simulink model "qbot_platform_obstacle_detection"  (R2023a)
settings: Solver=ode1  StartTime=0.0  StopTime=inf  FixedStep=1/30  RelTol=1e-3  EnableMultiTasking=on
InitFcn:
  | theta = linspace(pi/2, pi/4, 52);
  | theta_p = pi/2 - theta;
  | first = 1./cos(theta_p);
  | middle = first(end).*ones(1, 106);
  | last = flip(first);
  | 
  | zone = [first, middle, last]';
model workspace (MAT data in the model file):
  downCamStepSize = Simulink.Parameter
  downCamStepSize.Value = Simulink.data.Expression
  downCamStepSize.Value.ExpressionString = "qc_get_step_size*ceil(1/30/qc_get_step_size)"
  downCamStepSize.DataType = 'auto'
  downCamStepSize.Complexity = 'real'
  downCamStepSize.Dimensions = -1
  lidarStepSize = Simulink.Parameter
  lidarStepSize.Value = Simulink.data.Expression
  lidarStepSize.Value.ExpressionString = "qc_get_step_size*ceil(1/5/qc_get_step_size)"
  lidarStepSize.DataType = 'auto'
  lidarStepSize.Complexity = 'real'
  lidarStepSize.Dimensions = -1
  mainStepSize = Simulink.Parameter
  mainStepSize.Value = Simulink.data.Expression
  mainStepSize.Value.ExpressionString = "qc_get_step_size"
  mainStepSize.DataType = 'auto'
  mainStepSize.Complexity = 'real'
  mainStepSize.Dimensions = -1
  realSenseStepSize = Simulink.Parameter
  realSenseStepSize.Value = Simulink.data.Expression
  realSenseStepSize.Value.ExpressionString = "qc_get_step_size*ceil(1/30/qc_get_step_size)"
  realSenseStepSize.DataType = 'auto'
  realSenseStepSize.Complexity = 'real'
  realSenseStepSize.Dimensions = -1
undefined symbols (not defined in the file): Point, qc_get_step_size
libraries: quarc_library x12, simulink x2
settings Model: SimulationMode=external  ExtModeTrigDuration=10000  Creator=mbohra  LastModifiedBy=mbohra
settings SolverCC: AlgebraicLoopSolver=TrustRegion  PositivePriorityOrder=on
settings DataIOCC: ReturnWorkspaceOutputs=off
settings DebuggingCC: UnconnectedInputMsg=warning  UnconnectedOutputMsg=warning  UnconnectedLineMsg=warning  ArithmeticOperatorsInVariantConditions=warning
settings HardwareCC: ProdBitPerLong=64  ProdLargestAtomicInteger=LongLong  ProdLargestAtomicFloat=Double  ProdLongLongMode=on  ProdHWDeviceType=ARM Compatible->ARM 64-bit (LP64)
settings ModelReferenceCC: EnableRefExpFcnMdlSchedulingChecks=on
settings SFSimCC: SimUseLocalCustomCode=off  CustomCodeUndefinedFunction=UseInterfaceOnly
settings RTWCC: Description=QUARC Linux Raspberry Pi Arm64 Target (QBot Platform Alpha) Using Toolchain  SystemTargetFile=quarc_linux_pi_arm64.tlc  TemplateMakefile=quarc_default_tmf  RTWUseLocalCustomCode=off  Toolchain=QUARC linux_pi_arm64 | gmake (64-bit Windows)  BuildConfiguration=Faster Runs
settings CodeAppCC: StateflowObjectComments=on
settings STFCustomTargetCC: SystemTargetFile=quarc_linux_pi_arm64.tlc
settings GRTTargetCC: ParMdlRefBuildCompliant=off  CompOptLevelCompliant=off  CombineOutputUpdateFcns=off  MatFileLogging=off  CPPClassGenCompliant=off  GRTInterface=on  ExtMode=on  ExtModeMexFile=quarc_comm  ExtModeMexArgs='-w -d /tmp -uri %u','tcpip://192.168.2.80:17001'
settings ConfigComp: CovMetricSettings=dswe

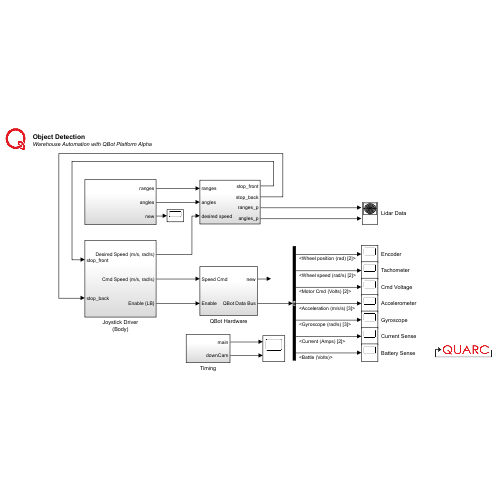
[thumbnail: Simulink's stored preview of the top-level diagram]
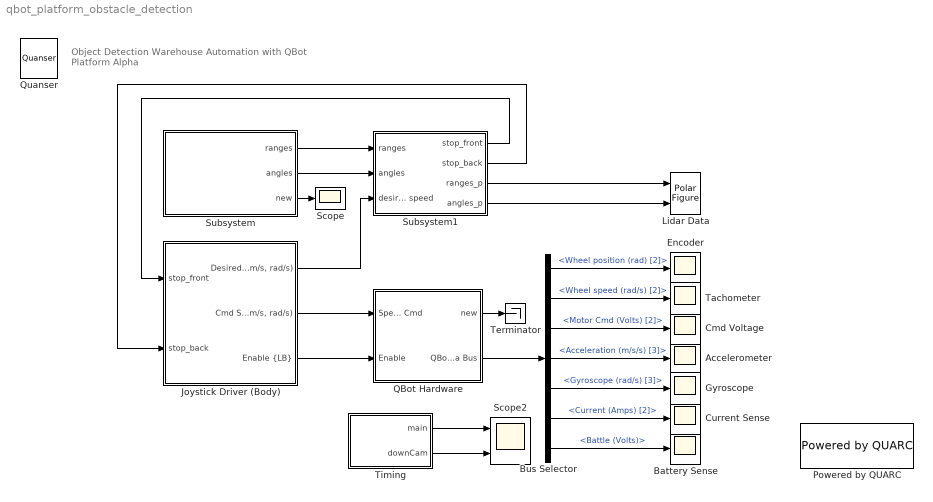
== system qbot_platform_obstacle_detection ==
  note: Object Detection
      | Warehouse Automation with QBot Platform Alpha
  Accelerometer : Scope
  Battery Sense : Scope
  Bus Selector : BusSelector  OutputSignals=Wheel position (rad) [2],Wheel speed (rad/s) [2],Motor Cmd (Volts) [2],Acceleration (m/s/s) [3],Gyroscope (rad/s) [3],Current (Amps) [2],Battle (Volts)
  Cmd Voltage : Scope
  Current Sense : Scope
  Encoder : Scope
  Gyroscope : Scope
  Joystick Driver (Body) : Subsystem
  Lidar Data : quarc_library/Sinks/Figures/Polar Figure  figure_mode=Use figure window  figure_tag=figure1  axes_tag=axes1  plot_mode=Frame-based  minimum_rho=0  maximum_rho=4  minimum_theta=0  maximum_theta=360  zero_location=top  direction=counterclockwise  buffer_size=1  update_rate=1  sample_time=-1  initial_position="962   50  958  973"  initial_visibility=off  line1_style=None  line1_width=0.5  line1_color=[0 0.4470 0.7410]  marker1=Point (.)  marker1_size=6  marker1_edge_color=[0 0.447059 0.741176]  marker1_face_color=[0 0.447059 0.741176]  line2_style=Solid line (-)  line2_width=0.5  line2_color=[0.85098 0.32549 0.0980392]  marker2=None  marker2_size=6  marker2_edge_color=[0.85098 0.32549 0.0980392]  marker2_face_color=[0.85098 0.32549 0.0980392]  line3_style=Solid line (-)  line3_width=0.5  line3_color=[0.929412 0.694118 0.12549]  marker3=None  marker3_size=6  marker3_edge_color=[0.929412 0.694118 0.12549]  marker3_face_color=[0.929412 0.694118 0.12549]  line4_style=Solid line (-)  line4_width=0.5  line4_color=[0.494118 0.184314 0.556863]  marker4=None  marker4_size=6  marker4_edge_color=[0.494118 0.184314 0.556863]  marker4_face_color=[0.494118 0.184314 0.556863]  line5_style=Solid line (-)  line5_width=0.5  line5_color=[0.466667 0.67451 0.188235]  marker5=None  marker5_size=6  marker5_edge_color=[0.466667 0.67451 0.188235]  marker5_face_color=[0.466667 0.67451 0.188235]
      settings: SourceProductName=QUARC Targets
  Powered by QUARC : quarc_library/Logos/Powered by QUARC
  QBot Hardware : Subsystem
  Quanser : quarc_library/Logos/Quanser
  Scope : Scope
  Scope2 : Scope  NumInputPorts=2
  Subsystem : Subsystem
  Subsystem1 : Subsystem
  Tachometer : Scope
  Terminator : Terminator
  Timing : Subsystem
  wires:
  Timing/1(main) -> Scope2/1
  Timing/2(downCam) -> Scope2/2
  QBot Hardware/2(QBot Data Bus) -> Bus Selector/1
  Bus Selector/1 -> Encoder/1  "<Wheel position (rad) [2]>"
  Bus Selector/3 -> Cmd Voltage/1  "<Motor Cmd (Volts) [2]>"
  Bus Selector/4 -> Accelerometer/1  "<Acceleration (m/s/s) [3]>"
  Bus Selector/6 -> Current Sense/1  "<Current (Amps) [2]>"
  Bus Selector/2 -> Tachometer/1  "<Wheel speed (rad/s) [2]>"
  Bus Selector/5 -> Gyroscope/1  "<Gyroscope (rad/s) [3]>"
  Bus Selector/7 -> Battery Sense/1  "<Battle (Volts)>"
  Joystick Driver (Body)/3("Enable {LB}") -> QBot Hardware/2(Enable)
  Joystick Driver (Body)/2("Cmd Speed (m/s, rad/s)") -> QBot Hardware/1(Speed Cmd)
  QBot Hardware/1(new) -> Terminator/1
  Subsystem/3(new) -> Scope/1
  Subsystem/1(ranges) -> Subsystem1/1(ranges)
  Subsystem/2(angles) -> Subsystem1/2(angles)
  Joystick Driver (Body)/1("Desired Speed (m/s, rad/s)") -> Subsystem1/3(desired speed)
  Subsystem1/3(ranges_p) -> Lidar Data/1
  Subsystem1/4(angles_p) -> Lidar Data/2
  Subsystem1/1(stop_front) -> Joystick Driver (Body)/1(stop_front)
  Subsystem1/2(stop_back) -> Joystick Driver (Body)/2(stop_back)

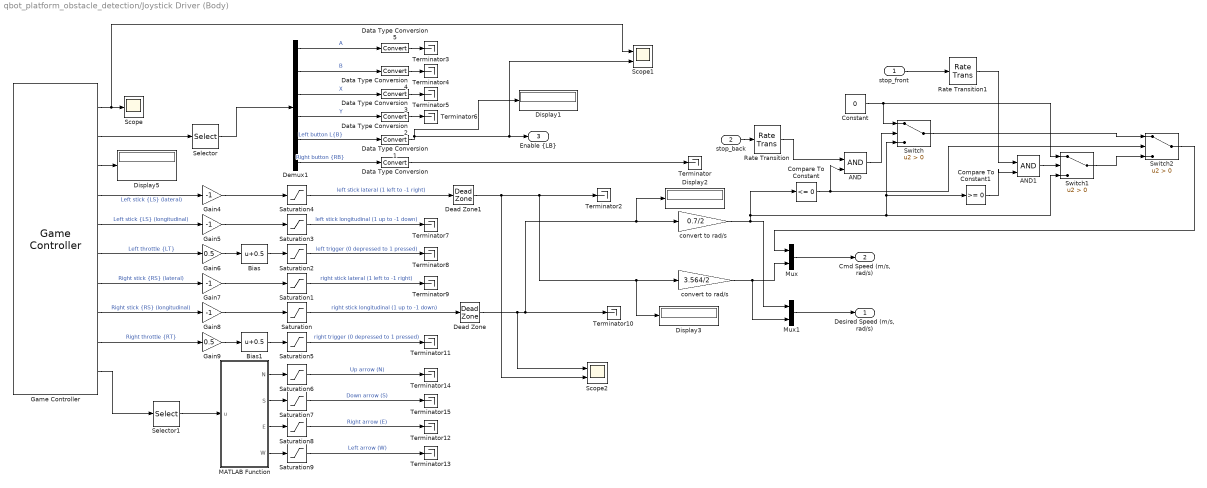
== system qbot_platform_obstacle_detection/Joystick Driver (Body) ==
  stop_front : Inport
  stop_back : Inport  Port=2
  AND : Logic  IconShape=distinctive  AllPortsSameDT=off  OutDataTypeStr=boolean
  AND1 : Logic  IconShape=distinctive  AllPortsSameDT=off  OutDataTypeStr=boolean
  Bias : Bias  Bias=0.5  SaturateOnIntegerOverflow=off
  Bias1 : Bias  Bias=0.5  SaturateOnIntegerOverflow=off
  Compare To Constant : simulink/Logic and Bit Operations/Compare To Constant  relop=<=  const=0  OutDataTypeStr=boolean
  Compare To Constant1 : simulink/Logic and Bit Operations/Compare To Constant  relop=>=  const=0  OutDataTypeStr=boolean
  Constant : Constant  Value=0
  Data Type Conversion{,1..5} (6 alike) : DataTypeConversion  SaturateOnIntegerOverflow=off  RndMeth=Floor
  Dead Zone : DeadZone  LowerValue=-0.05  UpperValue=0.05
  Dead Zone1 : DeadZone  LowerValue=-0.05  UpperValue=0.05
  Demux1 : Demux  Outputs=6
  Display{1..3,5} (4 alike) : Display
  Gain{4..5,7..8} (4 alike) : Gain  Gain=-1
  Gain6 : Gain  Gain=0.5
  Gain9 : Gain  Gain=0.5
  Game Controller : quarc_library/Devices/Peripherals/Target/Game Controller  controller=1  buffer_size=12  deadzone=[]  saturation=[]  sample_time=qc_get_step_size  auto_center=off  enabled=on
      settings: SourceProductName=QUARC Targets
  MATLAB Function : MATLAB Function  TreatAsAtomicUnit=on
  Mux : Mux  Inputs=2
  Mux1 : Mux  Inputs=2
  Rate Transition : RateTransition
  Rate Transition1 : RateTransition
  Saturation{,1,3..4} (4 alike) : Saturate  UpperLimit=1  LowerLimit=-1
  Saturation{2,5..9} (6 alike) : Saturate  UpperLimit=1  LowerLimit=0
  Scope : Scope
  Scope1 : Scope  NumInputPorts=2
  Scope2 : Scope  NumInputPorts=2
  Selector : Selector  InputPortWidth=32  IndexOptions=Index vector (dialog)  Indices=[1:6]  OutputSizes=1
  Selector1 : Selector  InputPortWidth=4  IndexOptions=Index vector (dialog)  Indices=1  OutputSizes=1
  Switch : Switch  Criteria=u2 > Threshold  SaturateOnIntegerOverflow=off  InputSameDT=off
  Switch1 : Switch  Criteria=u2 > Threshold  SaturateOnIntegerOverflow=off  InputSameDT=off
  Switch2 : Switch  Criteria=u2 > Threshold  SaturateOnIntegerOverflow=off  InputSameDT=off
  Terminator{,2..15} (15 alike) : Terminator
  convert to rad/s : Gain  Gain=0.7/2
  "convert to rad/s " : Gain  Gain=3.564/2
  "Desired Speed (m/s, rad/s)" : Outport
  "Cmd Speed (m/s, rad/s)" : Outport  Port=2
  "Enable {LB}" : Outport  Port=3
  wires:
  convert to rad/s/1 -> Mux1/1, Switch1/3, Switch/3, Compare To Constant1/1, Compare To Constant/1
  Mux/1 -> "Cmd Speed (m/s, rad/s)"/1
  Game Controller/1 -> Scope1/1, Scope/1
  Game Controller/2 -> Selector/1
  Game Controller/3 -> Display5/1
  Game Controller/4 -> Gain4/1  "Left stick {LS} (lateral)"
  Game Controller/5 -> Gain5/1  "Left stick {LS} (longitudinal)"
  Game Controller/6 -> Gain6/1  "Left throttle {LT}"
  Game Controller/7 -> Gain7/1  "Right stick {RS} (lateral)"
  Game Controller/8 -> Gain8/1  "Right stick {RS} (longitudinal)"
  Game Controller/9 -> Gain9/1  "Right throttle {RT}"
  Game Controller/10 -> Selector1/1
  Selector/1 -> Demux1/1
  Demux1/1 -> Data Type Conversion5/1  "A"
  Demux1/2 -> Data Type Conversion4/1  "B"
  Demux1/3 -> Data Type Conversion3/1  "X"
  Demux1/4 -> Data Type Conversion2/1  "Y"
  Demux1/5 -> Data Type Conversion1/1  "Left button L{B}"
  Demux1/6 -> Data Type Conversion/1  "Right button {RB}"
  Selector1/1 -> MATLAB Function/1(u)
  Gain6/1 -> Bias/1
  Gain9/1 -> Bias1/1
  Gain8/1 -> Saturation/1
  Gain7/1 -> Saturation1/1
  Gain5/1 -> Saturation3/1
  Gain4/1 -> Saturation4/1
  Bias/1 -> Saturation2/1
  Bias1/1 -> Saturation5/1
  Saturation4/1 -> Dead Zone1/1  "left stick lateral (1 left to -1 right)"
  Saturation3/1 -> Terminator7/1  "left stick longitudinal (1 up to -1 down)"
  Saturation2/1 -> Terminator8/1  "left trigger (0 depressed to 1 pressed)"
  Saturation1/1 -> Terminator9/1  "right stick lateral (1 left to -1 right)"
  Saturation/1 -> Dead Zone/1  "right stick longitudinal (1 up to -1 down)"
  Saturation5/1 -> Terminator11/1  "right trigger (0 depressed to 1 pressed)"
  MATLAB Function/1(N) -> Saturation6/1
  MATLAB Function/2(S) -> Saturation7/1
  MATLAB Function/3(E) -> Saturation8/1
  MATLAB Function/4(W) -> Saturation9/1
  Saturation6/1 -> Terminator14/1  "Up arrow (N)"
  Saturation7/1 -> Terminator15/1  "Down arrow (S)"
  Saturation8/1 -> Terminator12/1  "Right arrow (E)"
  Saturation9/1 -> Terminator13/1  "Left arrow (W)"
  Data Type Conversion1/1 -> Display1/1, Scope1/2, "Enable {LB}"/1
  Data Type Conversion2/1 -> Terminator6/1
  Data Type Conversion3/1 -> Terminator5/1
  Data Type Conversion4/1 -> Terminator4/1
  Data Type Conversion5/1 -> Terminator3/1
  Data Type Conversion/1 -> Terminator/1
  "convert to rad/s "/1 -> Mux1/2, Mux/2
  Dead Zone/1 -> Scope2/1, convert to rad/s/1, Display2/1, Terminator10/1
  Dead Zone1/1 -> Scope2/2, "convert to rad/s "/1, Display3/1, Terminator2/1
  stop_back/1 -> Rate Transition/1
  Compare To Constant/1 -> Switch2/2, AND/2
  AND/1 -> Switch/2
  Constant/1 -> Switch/1, Switch1/1
  Compare To Constant1/1 -> AND1/2
  stop_front/1 -> Rate Transition1/1
  AND1/1 -> Switch1/2
  Rate Transition/1 -> AND/1
  Rate Transition1/1 -> AND1/1
  Switch/1 -> Switch2/1
  Switch1/1 -> Switch2/3
  Switch2/1 -> Mux/1
  Mux1/1 -> "Desired Speed (m/s, rad/s)"/1

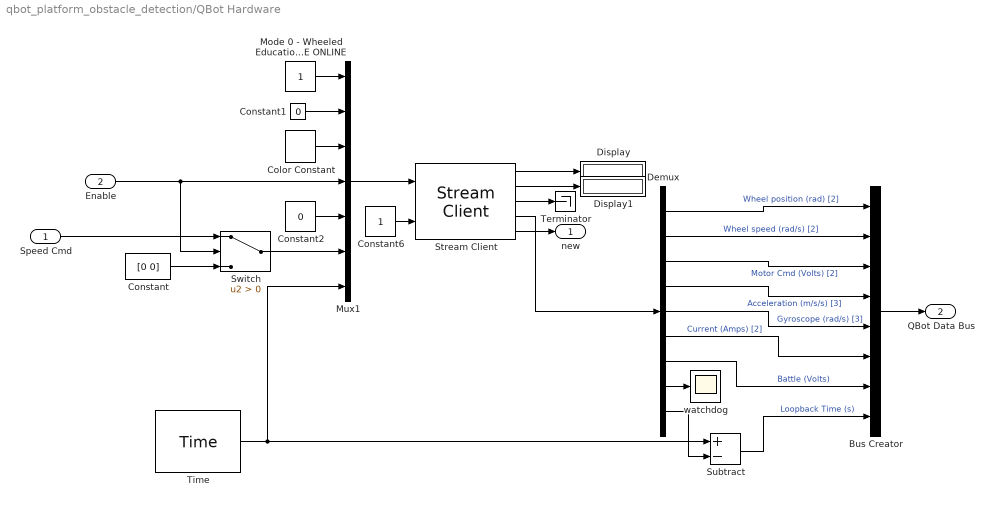
== system qbot_platform_obstacle_detection/QBot Hardware ==
  Speed Cmd : Inport
  Enable : Inport  Port=2
  Bus Creator : BusCreator  Inputs=8
  Color Constant : quarc_library/Sources/Signals/Color Constant  color=[0 1 1]
      settings: SourceProductName=QUARC Targets
  Constant : Constant  Value=[0 0]
  Constant1 : Constant  Value=0
  Constant2 : Constant  Value=0
  Constant6 : Constant
  Demux : Demux  Outputs=[2 2 2 3 3 2 1 1 1]
  Display : Display
  Display1 : Display
  Mode 0 - Wheeled Education Mode Mode 1 - Body Education Mode Mode 2 - Wheeled Research Mode Mode 3 - Body Research Mode DO NOT CHANGE ONLINE : Constant
  Mux1 : Mux  Inputs=7
  Stream Client : quarc_library/Communications/Basic/Stream Client  uri_source=Specify via dialog (do not evaluate)  uri=tcpip://localhost:18888  send_buffer_size=1460  receive_buffer_size=1460  byte_order=little endian (Intel - LSB first)  optimization=Minimum latency  send_options=Send most recent data  receive_options=Receive most recent data  default_value=zeros(17,1)  sample_time=qc_get_step_size  active=off  implementation=Use blocking I/O in a separate thread  send_fifo_size=1000  receive_fifo_size=1000  send_priority=0  receive_priority=0  send_dimensions=off  receive_dimensions=off  max_dimensions=-1  data_type=Inherited via back propagation  type_expr=BusObject
      settings: AttributesFormatString="\"tcpip://localhost:18888\""
  Subtract : Sum  Inputs=+-
  Switch : Switch  Criteria=u2 > Threshold  SaturateOnIntegerOverflow=off  InputSameDT=off
  Terminator : Terminator
  Time : quarc_library/Sources/Time/Time  time_source=Wall clock  sample_time=qc_get_step_size
  watchdog : Scope
  new : Outport
  QBot Data Bus : Outport  Port=2
  wires:
  Demux/2 -> Bus Creator/2  "Wheel speed (rad/s) [2]"
  Mode 0 - Wheeled Education Mode Mode 1 - Body Education Mode Mode 2 - Wheeled Research Mode Mode 3 - Body Research Mode DO NOT CHANGE ONLINE/1 -> Mux1/1
  Stream Client/3 -> Terminator/1
  Speed Cmd/1 -> Switch/1
  Stream Client/1 -> Display/1
  Constant6/1 -> Stream Client/2
  Stream Client/2 -> Display1/1
  Color Constant/1 -> Mux1/3
  Constant1/1 -> Mux1/2
  Demux/3 -> Bus Creator/3  "Motor Cmd (Volts) [2]"
  Mux1/1 -> Stream Client/1
  Stream Client/4 -> Demux/1
  Demux/1 -> Bus Creator/1  "Wheel position (rad) [2]"
  Stream Client/5 -> new/1
  Demux/7 -> Bus Creator/7  "Battle (Volts)"
  Demux/5 -> Bus Creator/5  "Gyroscope (rad/s) [3]"
  Demux/6 -> Bus Creator/6  "Current (Amps) [2]"
  Demux/9 -> Subtract/2
  Constant2/1 -> Mux1/5
  Demux/4 -> Bus Creator/4  "Acceleration (m/s/s) [3]"
  Enable/1 -> Switch/2, Mux1/4
  Time/1 -> Mux1/7, Subtract/1
  Bus Creator/1 -> QBot Data Bus/1
  Subtract/1 -> Bus Creator/8  "Loopback Time (s)"
  Demux/8 -> watchdog/1
  Switch/1 -> Mux1/6
  Constant/1 -> Switch/3

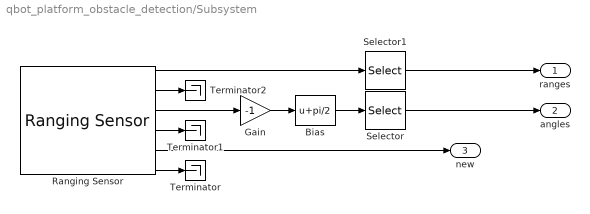
== system qbot_platform_obstacle_detection/Subsystem ==
  Bias : Bias  Bias=pi/2  SaturateOnIntegerOverflow=off
  Gain : Gain  Gain=-1
  Ranging Sensor : quarc_library/Devices/Third-Party/Sensors/Ranging Sensor  sensor_type=Leishen M10P LIDAR  uri=serial://localhost:0?baud='512000',word='8',parity='none',stop='1',flow='none',device='/dev/lidar'  ranging_distance=Short  timing_budget=0.033  measurement_period=0.0005  output_mode=Fixed-size output  samples_per_revolution=1680  max_distance=0.050  max_angle=5  sample_time=qc_get_step_size*3  show_versions=off  active=on
      settings: SourceProductName=QUARC Targets
  Selector : Selector  InputPortWidth=1680  IndexOptions=Index vector (dialog)  Indices=[1:4:1677]  OutputSizes=1
  Selector1 : Selector  InputPortWidth=1680  IndexOptions=Index vector (dialog)  Indices=[1:4:1677]  OutputSizes=1
  Terminator : Terminator
  Terminator1 : Terminator
  Terminator2 : Terminator
  ranges : Outport
  angles : Outport  Port=2
  new : Outport  Port=3
  wires:
  Ranging Sensor/3 -> Gain/1
  Selector/1 -> angles/1
  Bias/1 -> Selector/1
  Gain/1 -> Bias/1
  Ranging Sensor/1 -> Selector1/1
  Ranging Sensor/5 -> new/1
  Selector1/1 -> ranges/1
  Ranging Sensor/6 -> Terminator/1
  Ranging Sensor/4 -> Terminator1/1
  Ranging Sensor/2 -> Terminator2/1

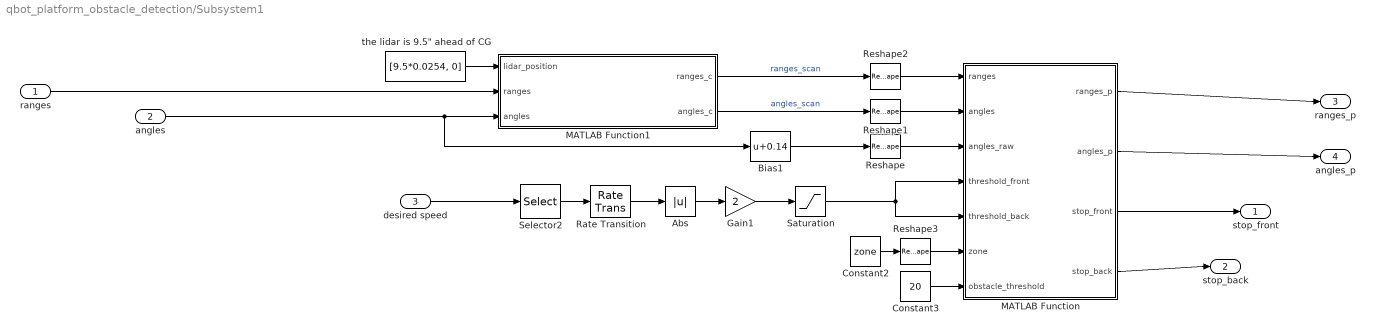
== system qbot_platform_obstacle_detection/Subsystem1 ==
  ranges : Inport
  angles : Inport  Port=2
  desired speed : Inport  Port=3
  Abs : Abs  SaturateOnIntegerOverflow=off
  Bias1 : Bias  Bias=0.14  SaturateOnIntegerOverflow=off
  Constant2 : Constant  Value=zone
  Constant3 : Constant  Value=20
  Gain1 : Gain  Gain=2
  MATLAB Function : MATLAB Function  TreatAsAtomicUnit=on
  MATLAB Function1 : MATLAB Function  TreatAsAtomicUnit=on
  Rate Transition : RateTransition
  Reshape{,1..3} (4 alike) : Reshape  OutputDimensionality=Column vector (2-D)
  Saturation : Saturate  UpperLimit=1  LowerLimit=0.5
  Selector2 : Selector  InputPortWidth=2  IndexOptions=Index vector (dialog)  Indices=1  OutputSizes=1
  "the lidar is 9.5\" ahead of CG" : Constant  Value=[9.5*0.0254, 0]  SampleTime=qc_get_step_size*3
  stop_front : Outport
  stop_back : Outport  Port=2
  ranges_p : Outport  Port=3
  angles_p : Outport  Port=4
  wires:
  Gain1/1 -> Saturation/1
  Constant2/1 -> Reshape3/1
  Selector2/1 -> Rate Transition/1
  "the lidar is 9.5\" ahead of CG"/1 -> MATLAB Function1/1(lidar_position)
  Constant3/1 -> MATLAB Function/7(obstacle_threshold)
  Reshape3/1 -> MATLAB Function/6(zone)
  Saturation/1 -> MATLAB Function/5(threshold_back), MATLAB Function/4(threshold_front)
  Abs/1 -> Gain1/1
  angles/1 -> Bias1/1, MATLAB Function1/3(angles)
  Reshape2/1 -> MATLAB Function/1(ranges)
  MATLAB Function1/2(angles_c) -> Reshape1/1  "angles_scan"
  MATLAB Function1/1(ranges_c) -> Reshape2/1  "ranges_scan"
  Rate Transition/1 -> Abs/1
  Bias1/1 -> Reshape/1
  ranges/1 -> MATLAB Function1/2(ranges)
  Reshape1/1 -> MATLAB Function/2(angles)
  Reshape/1 -> MATLAB Function/3(angles_raw)
  MATLAB Function/3(stop_front) -> stop_front/1
  MATLAB Function/2(angles_p) -> angles_p/1
  MATLAB Function/1(ranges_p) -> ranges_p/1
  MATLAB Function/4(stop_back) -> stop_back/1
  desired speed/1 -> Selector2/1

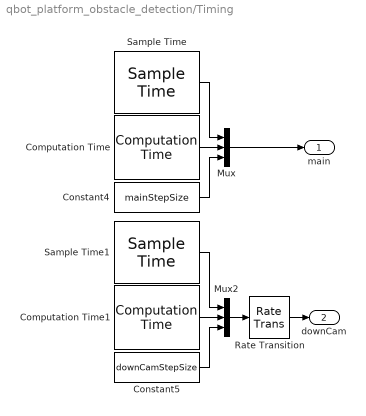
== system qbot_platform_obstacle_detection/Timing ==
  Computation Time : quarc_library/Sources/Time/Computation Time  sample_time=mainStepSize  use_model=on  use_cpu_time=off
  Computation Time1 : quarc_library/Sources/Time/Computation Time  sample_time=downCamStepSize  use_model=on  use_cpu_time=off
  Constant4 : Constant  Value=mainStepSize
  Constant5 : Constant  Value=downCamStepSize
  Mux : Mux  Inputs=3
  Mux2 : Mux  Inputs=3
  Rate Transition : RateTransition
  Sample Time : quarc_library/Sources/Time/Sample Time  Priority=-99  sample_time=mainStepSize
  Sample Time1 : quarc_library/Sources/Time/Sample Time  Priority=-99  sample_time=downCamStepSize
  main : Outport
  downCam : Outport  Port=2
  wires:
  Constant5/1 -> Mux2/3
  Computation Time/1 -> Mux/2
  Sample Time/1 -> Mux/1
  Sample Time1/1 -> Mux2/1
  Computation Time1/1 -> Mux2/2
  Constant4/1 -> Mux/3
  Mux2/1 -> Rate Transition/1
  Rate Transition/1 -> downCam/1
  Mux/1 -> main/1

== matlab function qbot_platform_obstacle_detection/Subsystem1/MATLAB Function ==
  data: ranges_p output; angles_p output; ranges input; angles input; angles_raw input; stop_front output; stop_back output; threshold_front input; threshold_back input; zone input; obstacle_threshold input
function [ranges_p, angles_p, stop_front, stop_back] = detect_obstacles(ranges, angles, angles_raw, threshold_front, threshold_back, zone, obstacle_threshold)

angles_p = [angles; angles_raw];
ranges_p = [ranges; ranges];

ranges_p(421:630) = threshold_front.*zone/sqrt(2);
ranges_p(631:840) = threshold_back.*zone/sqrt(2);

stop_front = sum((ranges(1:210) > 0.25) .* (ranges(1:210) < ranges_p(421:630))) > obstacle_threshold;
stop_back = sum((ranges(211:420) > 0.25) .* (ranges(211:420) < ranges_p(631:840))) > obstacle_threshold;
     
end

== matlab function qbot_platform_obstacle_detection/Joystick Driver (Body)/MATLAB Function ==
  data: u input; N output; S output; E output; W output
function [N, S, E, W] = fcn(u)

N = 0;
S = 0;
E = 0;
W = 0;

switch u
    case 0
        N = 1;
    case 3.142
        S = 1;
    case 4.712
        W = 1;
    case 1.571
        E = 1;
    case 3.927
        S = 1;
        W = 1;
    case 2.356
        S = 1;
        E = 1;
    case 0.7854
        N = 1;
        E = 1;
    case 5.498
        N = 1;
        W = 1;
end

== matlab function qbot_platform_obstacle_detection/Subsystem1/MATLAB Function1 ==
  data: lidar_position input; ranges input; ranges_c output; angles input; angles_c output
function [ranges_c,angles_c] = correct_lidar(lidar_position, ranges,angles)

x = ranges.*cos(angles) + lidar_position(1);
y = ranges.*sin(angles) + lidar_position(2);

ranges_c = sqrt(x.^2 + y.^2);
angles_c = atan2(y, x);

end
